simulink model "obsluga_analogow"  (Simulink 8.4)
settings: Solver=ode45  StartTime=0.0  StopTime=10.0  RelTol=1e-3
settings Model: Creator=Michal  LastModifiedBy=Michal
settings DataIOCC: SignalLoggingSaveFormat=Dataset
settings OptimizationCC: ExpressionDepthLimit=128
settings DebuggingCC: UnderspecifiedInitializationDetection=Simplified  MergeDetectMultiDrivingBlocksExec=error  FcnCallInpInsideContextMsg=EnableAllAsError  StateNameClashWarn=none
settings GRTTargetCC: CombineOutputUpdateFcns=on  GRTInterface=off
settings ConfigComp: Description=PLC Coder Custom Configuration Component  PLC_TargetIDE=pcworx60  PLC_GenerateReport=off

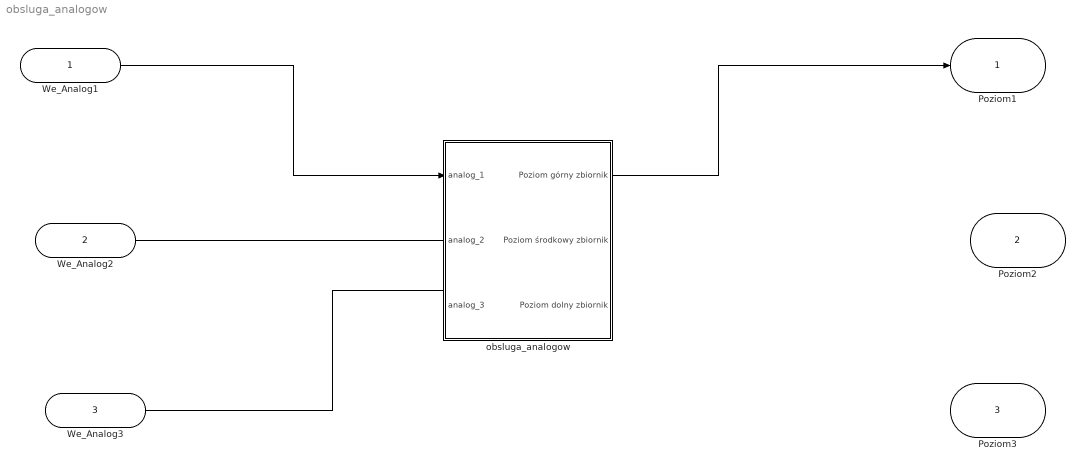
== system obsluga_analogow ==
  We_Analog1 : Inport
  We_Analog2 : Inport  Port=2
  We_Analog3 : Inport  Port=3
  obsluga_analogow : Subsystem  TreatAsAtomicUnit=on
  Poziom1 : Outport
  Poziom2 : Outport  Port=2
  Poziom3 : Outport  Port=3
  wires:
  We_Analog1/1 -> obsluga_analogow/1(analog_1)
  We_Analog2/1 -> ?
  We_Analog3/1 -> ?
  obsluga_analogow/1(Poziom górny zbiornik) -> Poziom1/1
  ? -> Poziom2/1
  ? -> Poziom3/1

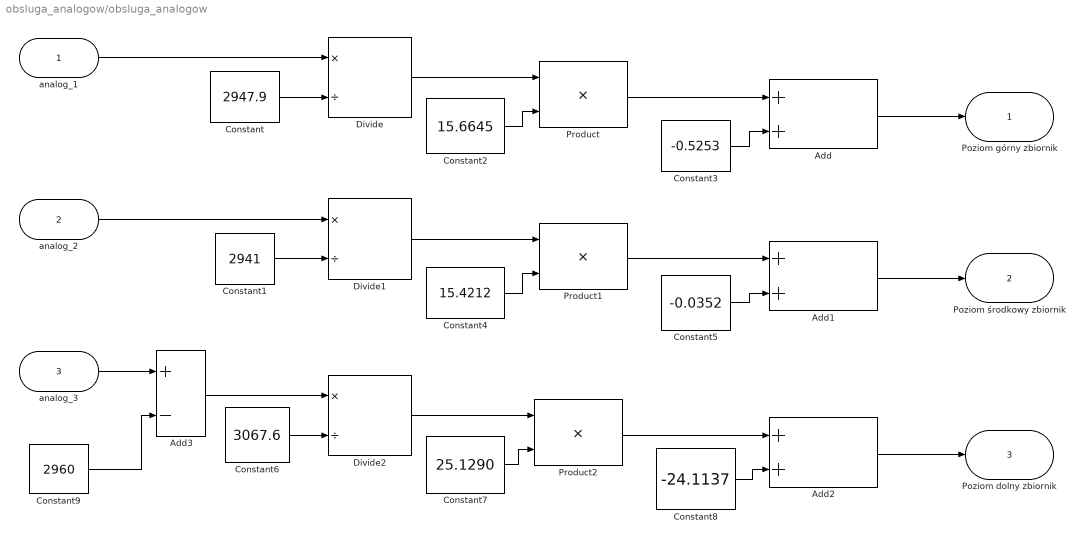
== system obsluga_analogow/obsluga_analogow ==
  analog_1 : Inport  OutDataTypeStr=single
  analog_2 : Inport  Port=2  OutDataTypeStr=single
  analog_3 : Inport  Port=3  OutDataTypeStr=single
  Add : Sum
  Add1 : Sum
  Add2 : Sum
  Add3 : Sum  Inputs=+-
  Constant : Constant  Value=2947.9  OutDataTypeStr=single
  Constant1 : Constant  Value=2941  OutDataTypeStr=single
  Constant2 : Constant  Value=15.6645  OutDataTypeStr=single
  Constant3 : Constant  Value=-0.5253  OutDataTypeStr=single
  Constant4 : Constant  Value=15.4212  OutDataTypeStr=single
  Constant5 : Constant  Value=-0.0352  OutDataTypeStr=single
  Constant6 : Constant  Value=3067.6  OutDataTypeStr=single
  Constant7 : Constant  Value=25.1290  OutDataTypeStr=single
  Constant8 : Constant  Value=-24.1137  OutDataTypeStr=single
  Constant9 : Constant  Value=2960  OutDataTypeStr=single
  Divide : Product  Inputs=*/
  Divide1 : Product  Inputs=*/
  Divide2 : Product  Inputs=*/
  Product : Product
  Product1 : Product
  Product2 : Product
  Poziom górny zbiornik : Outport
  Poziom środkowy zbiornik : Outport  Port=2
  Poziom dolny zbiornik : Outport  Port=3
  wires:
  analog_1/1 -> Divide/1
  Constant4/1 -> Product1/2
  Product1/1 -> Add1/1
  Constant5/1 -> Add1/2
  Divide1/1 -> Product1/1
  Add1/1 -> Poziom środkowy zbiornik/1
  Constant6/1 -> Divide2/2
  Add2/1 -> Poziom dolny zbiornik/1
  Divide2/1 -> Product2/1
  Product2/1 -> Add2/1
  Constant7/1 -> Product2/2
  Constant8/1 -> Add2/2
  Divide/1 -> Product/1
  Add/1 -> Poziom górny zbiornik/1
  Constant2/1 -> Product/2
  Product/1 -> Add/1
  Constant/1 -> Divide/2
  Constant3/1 -> Add/2
  Constant1/1 -> Divide1/2
  analog_3/1 -> Add3/1
  Constant9/1 -> Add3/2
  analog_2/1 -> Divide1/1
  Add3/1 -> Divide2/1
